simulink model "helicopter_2DOF"  (R2026a)
settings: Solver=VariableStepAuto  StopTime=25
values from neighbouring files (symbols this model uses):
  act = getBaseVariable('act')    [run_simulink_simulations.m]
  aero = struct    [run_simulink_simulations.m]
  alpha0 = deg2rad(15)    [build_uncertain_linear_model.m]    (also in init.m; run_simulink_simulations.m = evalin('base','alpha0'))
  Aobs = A - Ke*Cmeas    [LQG_2DOF_Synthesis.m]    (also in PIDcomp_decoupler_sensitivity.m; run_simulink_simulations.m)
  beta0 = deg2rad(20)    [build_uncertain_linear_model.m]    (also in init.m; run_simulink_simulations.m = evalin('base','beta0'))
  Bobs = [B Ke]    [LQG_2DOF_Synthesis.m]    (also in PIDcomp_decoupler_sensitivity.m; run_simulink_simulations.m)
  Cobs = eye(size(A))    [LQG_2DOF_Synthesis.m]    (also in PIDcomp_decoupler_sensitivity.m; run_simulink_simulations.m)
  Ddec_phys = [0.00367730883727  -0.0180750563026; -0.000204187403773  0.138403763822]    [HINF_controllers.mat]    (also in HINF_synthesis.m = Du *      Ddec_scaled *      Du_inv)
  delta_plant = zeros(7,1)    [init.m]
  denFalpha = [1 28.9710633828]    [HINF_controllers.mat]
  denFbeta = [1 116.132169803]    [HINF_controllers.mat]
  Dobs = zeros(size(A,1), size(B,2) + size(Cmeas,1))    [LQG_2DOF_Synthesis.m]    (also in PIDcomp_decoupler_sensitivity.m = zeros(size(A,1),size(B,2)+size(Cmeas,1)); run_simulink_simulations.m = zeros(size(A,1),size(B,2)+size(Cmeas,1)))
  g = 9.81    [build_uncertain_linear_model.m]
  HINF_controller_id = 3    [init.m]
  Hy = (Jsensor.'*Vinv*Jsensor) \      (Jsensor.'*Vinv)    [HINF_setup.m]    (also in HINF_setup.mat = [0.105532740103  0  0; 0  -0.00735527189948  -0.020208443457; RAS_vectorized.m = (Jsensor.'*Vinv*Jsensor) \ (Jsensor.'*Vinv))
  Hy_LQG = [0.105532740103  0  0; 0  -0.00735527189948  -0.0202084434578]    [LQG_2DOF_Controllers.mat]    (also in LQG_2DOF_Synthesis.m = (Jsensor.'*Vinv*Jsensor) \      (Jsensor.'*Vinv))
  K_hinfsyn = minreal(          Du *          K_hinfsyn_scaled *          Dy_inv,          1e-7)    [HINF_synthesis.m]
  K_LQG = ss(      Ac_LQG,      Bc_LQG,      Cc_LQG,      Dc_LQG)    [LQG_2DOF_Synthesis.m]
  K_mix = minreal(          Du *          K_mix_scaled *          Dy_inv,          1e-7)    [HINF_synthesis.m]
  K_mu = minreal(          Du *          K_mu_scaled *          Dy_inv,          1e-7)    [MU_synthesis.m]
  Kalpha_tuned = pid(          alphaScaledToPhys *          Kalpha_tuned_scaled.Kp,          alphaScaledToPhys *          Kalpha_tuned_scaled.Ki,          alphaScaledToPhys *          Kalpha_tuned_scaled.Kd,          Kalpha_tuned_scaled.Tf)    [HINF_synthesis.m]
  Kbeta_tuned = pid(          betaScaledToPhys *          Kbeta_tuned_scaled.Kp,          betaScaledToPhys *          Kbeta_tuned_scaled.Ki,          betaScaledToPhys *          Kbeta_tuned_scaled.Kd,          Kbeta_tuned_scaled.Tf)    [HINF_synthesis.m]
  Ki_LQGI = [-6.12353410994  -0.048270119194; 0.0482701191938  -6.12353410994]    [LQG_2DOF_Controllers.mat]    (also in LQG_2DOF_Synthesis.m = Kaug_LQI(:,n+1:end))
  Kx_LQGI = [2.67945787682 0.0236091239115 4.27147445601 0.0421494721099 7.37552374356 0.124215129254 0.0236091239115 3.00325151028 0.0375549932522 4.81803854156 0.0741131674737 8.79398804244 ... (20 elements, 2x10)]    [LQG_2DOF_Controllers.mat]    (also in LQG_2DOF_Synthesis.m = Kaug_LQI(:,1:n))
  LQG_controller_id = 1    [init.m]
  LQG_plant_id = 1    [init.m]
  numFalpha = [5.51938404497 96.5040578252]    [HINF_controllers.mat]
  numFbeta = [0.20657402382 68.2554624776]    [HINF_controllers.mat]
  P_nominal_ext = ss(P_uncertain_ext.NominalValue)    [build_uncertain_linear_model.m]
  q0 = [alpha0; beta0]    [init.m]
  qdot0 = [0; 0]    [init.m]
  ref = struct    [run_simulink_simulations.m]
  Robust_plant_id = 2    [init.m]
  sensor = getBaseVariable('sensor')    [run_simulink_simulations.m]
  u0 = u0_nominal    [build_uncertain_linear_model.m]    (also in init.m = E0 \ [)
  x0 = [ ... (first row only)    [build_uncertain_linear_model.m]    (also in init.m = [alpha0; 0; beta0; 0])
  xhat0 = zeros(size(A,1),1)    [LQG_2DOF_Synthesis.m]    (also in PIDcomp_decoupler_sensitivity.m; run_simulink_simulations.m)
  y0_sensor = [ ... (first row only)    [HINF_setup.m]    (also in HINF_setup.mat = [2.53901483246 43.6957068665 -15.9039366646]; LQG_2DOF_Controllers.mat = [2.53901483246 43.6957068665 -15.9039366646]; LQG_2DOF_Synthesis.m; RAS_vectorized.m)
undefined symbols (not defined in the file or in its folder): params
libraries: simulink x4, slpidlib x2, cstblocks_lti x2, RCTblocks x2
settings Model: Creator=bonci  LastModifiedBy=giggi
settings DebuggingCC: UnderSpecifiedDimensionMsg=warning

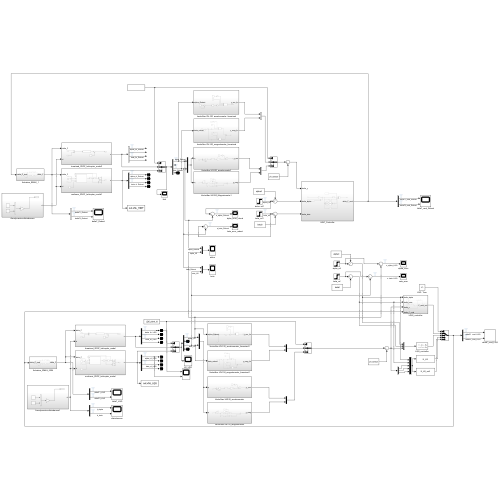
[thumbnail: Simulink's stored preview of the top-level diagram]
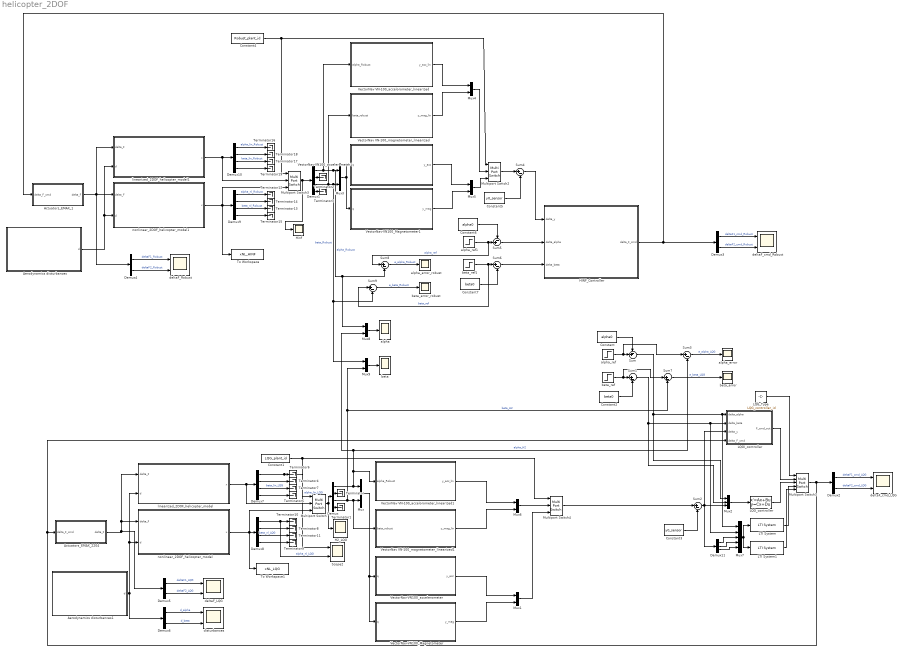
== system helicopter_2DOF ==
  Actuators_EMAX_1 : Subsystem
  Actuators_EMAX_2204 : Subsystem
  Aerodynamics disturbances : Subsystem
  Aerodynamics disturbances1 : Subsystem
  Constant : Constant  Value=alpha0
  Constant1 : Constant  Value=LQG_plant_id
  Constant2 : Constant  Value=beta0
  Constant3 : Constant  Value=y0_sensor
  Constant4 : Constant  Value=Robust_plant_id
  Constant5 : Constant  Value=y0_sensor
  Constant6 : Constant  Value=alpha0
  Constant7 : Constant  Value=beta0
  Demux{,1,7..10} (6 alike) : Demux
  Demux11 : Demux  Outputs=3
  Demux{2..6} (5 alike) : Demux  Outputs=2
  H2_LQG : Scope
      settings: ActiveDisplayYMinimum=0.24953416869226661  ActiveDisplayYMaximum=0.36288471920080412
  HINF_Controller : Subsystem
  Hinf : Scope
      settings: ActiveDisplayYMinimum=0.24925633700219857  ActiveDisplayYMaximum=0.36252454674659934
  LQGI_controller : Subsystem
  LQG_Type : Constant  Value=LQG_controller_id
  LQG_controller : StateSpace  A=K_LQG.A  B=K_LQG.B  C=K_LQG.C  D=K_LQG.D  InitialCondition=zeros(size(K_LQG.A,1),1)
  LTI System : cstblocks_lti/LTI System  sys=K_H2  IC=[]  PadeOrder=0
      settings: LibrarySourceBlock=cstblocks/LTI System
  LTI System1 : cstblocks_lti/LTI System  sys=K_H2_soft  IC=[]  PadeOrder=0
      settings: LibrarySourceBlock=cstblocks/LTI System
  Multiport Switch{,2..4} (4 alike) : MultiPortSwitch  Inputs=2  SaturateOnIntegerOverflow=off  InputSameDT=off
  Multiport Switch1 : MultiPortSwitch  Inputs=4  SaturateOnIntegerOverflow=off  InputSameDT=off
  Mux{,1,3..6,8..9} (8 alike) : Mux  Inputs=2
  Mux2 : Mux  Inputs=3
  Mux7 : Mux  Inputs=5
  Scope2 : Scope  NumInputPorts=2
      settings: ActiveDisplayYMinimum=0.25286399867414605  ActiveDisplayYMaximum=0.34221788992417967  DataLoggingVariableName=ScopeData11
  Sum : Sum  Inputs=-+|
  Sum{1..4,6..9} (8 alike) : Sum  Inputs=|+-
  Sum5 : Sum  Inputs=-+|
  Terminator{,1..19} (20 alike) : Terminator
  To Workspace : ToWorkspace  VariableName=xNL_HINF  SaveFormat=Timeseries  SampleTime=-1
  To Workspace1 : ToWorkspace  VariableName=xNL_LQG  SaveFormat=Timeseries  SampleTime=-1
  VectorNav VN-100_accelorometer_linearized : Subsystem
  VectorNav VN-100_accelorometer_linearized1 : Subsystem
  VectorNav VN-100_magnetometer_linearized : Subsystem
  VectorNav VN-100_magnetometer_linearized1 : Subsystem
  VectorNav-VN100_Magnetometer : Subsystem
  VectorNav-VN100_Magnetometer1 : Subsystem
  VectorNav-VN100_accelerometer : Subsystem
  VectorNav-VN100_accelerometer1 : Subsystem
  alpha : Scope
      settings: ActiveDisplayYMinimum=0.25090839242771618  ActiveDisplayYMaximum=0.2720900672525749  DataLoggingVariableName=ScopeData12
  alpha_error : Scope
      settings: DataLoggingVariableName=ScopeData2
  alpha_error_robust : Scope
      settings: DataLoggingVariableName=ScopeData4
  alpha_ref : Step  Time=ref.alpha.time  InitialValue=ref.alpha.initial  FinalValue=ref.alpha.final  SampleTime=0
  alpha_ref1 : Step  Time=ref.alpha.time  InitialValue=ref.alpha.initial  FinalValue=ref.alpha.final  SampleTime=0
  beta : Scope
      settings: ActiveDisplayYMinimum=0.33140553496326319  ActiveDisplayYMaximum=0.36028063841557784  DataLoggingVariableName=ScopeData13
  beta_error : Scope
      settings: ActiveDisplayYMinimum=-0.017727079570451457  ActiveDisplayYMaximum=0.0030981168879630895  DataLoggingVariableName=ScopeData3
  beta_error_robust : Scope
      settings: DataLoggingVariableName=ScopeData5
  beta_ref : Step  Time=ref.beta.time  InitialValue=ref.beta.initial  FinalValue=ref.beta.final  SampleTime=0
  beta_ref1 : Step  Time=ref.beta.time  InitialValue=ref.beta.initial  FinalValue=ref.beta.final  SampleTime=0
  deltaF_LQG : Scope  NumInputPorts=2
      settings: DataLoggingVariableName=ScopeData9
  deltaF_Robust : Scope  NumInputPorts=2
      settings: DataLoggingVariableName=ScopeData8
  deltaF_cmd_LQG : Scope  NumInputPorts=2
      settings: ActiveDisplayYMinimum=-6.7119063745859271E-6  ActiveDisplayYMaximum=6.008697179895143E-5  DataLoggingVariableName=ScopeData6
  deltaF_cmd_Robust : Scope  NumInputPorts=2
      settings: ActiveDisplayYMinimum=-5.0521969284629318E-5  ActiveDisplayYMaximum=0.00043770968760487613  DataLoggingVariableName=ScopeData7
  disturbances : Scope  NumInputPorts=2
      settings: DataLoggingVariableName=ScopeData10
  linearized_2DOF_helicopter_model : Subsystem
  linearized_2DOF_helicopter_model1 : Subsystem
  nonlinear_2DOF_helicopter_model : Subsystem
  nonlinear_2DOF_helicopter_model1 : Subsystem
  wires:
  nonlinear_2DOF_helicopter_model/1(x) -> Demux8/1, To Workspace1/1, Multiport Switch/3
  linearized_2DOF_helicopter_model/1(x) -> Multiport Switch/2, Demux7/1
  Constant1/1 -> Multiport Switch4/1, Multiport Switch/1
  Multiport Switch/1 -> Demux/1, H2_LQG/1
  VectorNav-VN100_accelerometer/1(y_acc) -> Mux1/1
  VectorNav-VN100_Magnetometer/1(y_mag) -> Mux1/2
  Demux/1 -> VectorNav VN-100_accelorometer_linearized1/1(alpha_Robust), Sum3/2, Mux8/2, Mux/1  "alpha_H2"
  Demux/3 -> Mux9/2, Sum7/2, VectorNav VN-100_magnetometer_linearized1/1(bata_robust), Mux/2  "beta_H2"
  Mux/1 -> VectorNav-VN100_Magnetometer/1(q), VectorNav-VN100_accelerometer/1(q)
  Demux/2 -> Terminator/1
  Demux/4 -> Terminator1/1
  alpha_ref/1 -> Sum3/1, Sum/2
  beta_ref/1 -> Sum7/1, Sum1/1
  Constant/1 -> Sum/1
  Constant2/1 -> Sum1/2
  Constant3/1 -> Sum2/2
  Sum/1 -> Mux7/1, LQGI_controller/1(delta_alpha), Mux2/1
  Mux2/1 -> LQG_controller/1
  LQG_controller/1 -> Multiport Switch1/3
  LQG_Type/1 -> Multiport Switch1/1
  Multiport Switch1/1 -> LQGI_controller/4(delta_F_cmd), Actuators_EMAX_2204/1(delta_F_cmd), Demux2/1
  LQGI_controller/1(F_cmd_out) -> Multiport Switch1/2
  Constant5/1 -> Sum4/2
  VectorNav-VN100_accelerometer1/1(y_acc) -> Mux5/1
  Demux1/1 -> VectorNav VN-100_accelorometer_linearized/1(alpha_Robust), Mux8/1, Sum8/2, Mux3/1  "alpha_Robust"
  VectorNav-VN100_Magnetometer1/1(y_mag) -> Mux5/2
  Mux3/1 -> VectorNav-VN100_Magnetometer1/1(q), VectorNav-VN100_accelerometer1/1(q)
  Demux1/2 -> Terminator2/1
  Demux1/4 -> Terminator3/1
  Demux1/3 -> VectorNav VN-100_magnetometer_linearized/1(bata_robust), Mux3/2, Mux9/1, Sum9/2  "beta_Robust"
  Constant4/1 -> Multiport Switch3/1, Multiport Switch2/1
  Multiport Switch3/1 -> Demux1/1, Hinf/1
  linearized_2DOF_helicopter_model1/1(x) -> Demux10/1, Multiport Switch3/2
  Constant6/1 -> Sum5/1
  alpha_ref1/1 -> Sum8/1, Sum5/2  "alpha_ref"
  beta_ref1/1 -> Sum9/1, Sum6/1  "beta_ref"
  Constant7/1 -> Sum6/2
  Sum4/1 -> HINF_Controller/1(delta_y)
  Sum5/1 -> HINF_Controller/2(delta_alpha)
  Sum6/1 -> HINF_Controller/3(delta_beta)
  Aerodynamics disturbances/1(d) -> linearized_2DOF_helicopter_model1/2(d), nonlinear_2DOF_helicopter_model1/2(d)
  Sum3/1 -> alpha_error/1  "e_alpha_LQG"
  Sum1/1 -> LQGI_controller/2(delta_beta), Mux7/2, Mux2/2
  Sum7/1 -> beta_error/1  "e_beta_LQG"
  Sum8/1 -> alpha_error_robust/1  "e_alpha_Robust"
  Sum9/1 -> beta_error_robust/1  "e_beta_Robust"
  Demux2/1 -> deltaF_cmd_LQG/1  "deltaF1_cmd_LQG"
  Demux2/2 -> deltaF_cmd_LQG/2  "deltaF2_cmd_LQG"
  Demux3/2 -> deltaF_cmd_Robust/2  "deltaF2_cmd_Robust"
  Demux3/1 -> deltaF_cmd_Robust/1  "deltaF1_cmd_Robust"
  HINF_Controller/1(delta_F_cmd) -> Demux3/1, Actuators_EMAX_1/1(delta_F_cmd)
  Actuators_EMAX_1/1(delta_F) -> nonlinear_2DOF_helicopter_model1/1(delta_F), linearized_2DOF_helicopter_model1/1(delta_F), Demux4/1
  Demux4/1 -> deltaF_Robust/1  "deltaF1_Robust"
  Demux4/2 -> deltaF_Robust/2  "deltaF2_Robust"
  Demux5/1 -> deltaF_LQG/1  "deltaF1_LQG"
  Demux5/2 -> deltaF_LQG/2  "deltaF2_LQG"
  Actuators_EMAX_2204/1(delta_F) -> Demux5/1, nonlinear_2DOF_helicopter_model/1(delta_F), linearized_2DOF_helicopter_model/1(delta_F)
  Demux6/2 -> disturbances/2  "d_beta"
  Aerodynamics disturbances1/1(d) -> Demux6/1, nonlinear_2DOF_helicopter_model/2(d), linearized_2DOF_helicopter_model/2(d)
  Demux6/1 -> disturbances/1  "d_alpha"
  Demux7/4 -> Terminator5/1
  Demux7/1 -> Scope2/1, Terminator6/1  "alpha_lin_LQG"
  Demux7/3 -> Terminator7/1  "beta_lin_LQG"
  Demux7/2 -> Terminator4/1
  Demux8/1 -> Scope2/2, Terminator10/1  "alpha_nl_LQG"
  Demux8/2 -> Terminator8/1
  Demux8/3 -> Terminator11/1  "beta_nl_LQG"
  Demux8/4 -> Terminator9/1
  Demux9/4 -> Terminator15/1
  Demux9/3 -> Terminator13/1  "beta_nl_Robust"
  nonlinear_2DOF_helicopter_model1/1(x) -> Demux9/1, To Workspace/1, Multiport Switch3/3
  Demux9/1 -> Terminator12/1  "alpha_nl_Robust"
  Demux9/2 -> Terminator14/1
  Demux10/3 -> Terminator17/1  "beta_lin_Robust"
  Demux10/4 -> Terminator19/1
  Demux10/1 -> Terminator16/1  "alpha_lin_Robust"
  Demux10/2 -> Terminator18/1
  Mux5/1 -> Multiport Switch2/3
  Multiport Switch2/1 -> Sum4/1
  Mux1/1 -> Multiport Switch4/3
  Multiport Switch4/1 -> Sum2/1
  VectorNav VN-100_magnetometer_linearized/1(y_mag_lin) -> Mux4/2
  VectorNav VN-100_accelorometer_linearized/1(y_acc_lin) -> Mux4/1
  Mux4/1 -> Multiport Switch2/2
  VectorNav VN-100_accelorometer_linearized1/1(y_acc_lin) -> Mux6/1
  VectorNav VN-100_magnetometer_linearized1/1(y_mag_lin) -> Mux6/2
  Mux6/1 -> Multiport Switch4/2
  Sum2/1 -> Demux11/1, LQGI_controller/3(delta_y), Mux2/3
  Demux11/1 -> Mux7/3
  Demux11/2 -> Mux7/4
  Demux11/3 -> Mux7/5
  Mux7/1 -> LTI System1/1, LTI System/1
  LTI System/1 -> Multiport Switch1/4
  LTI System1/1 -> Multiport Switch1/5
  Mux8/1 -> alpha/1
  Mux9/1 -> beta/1

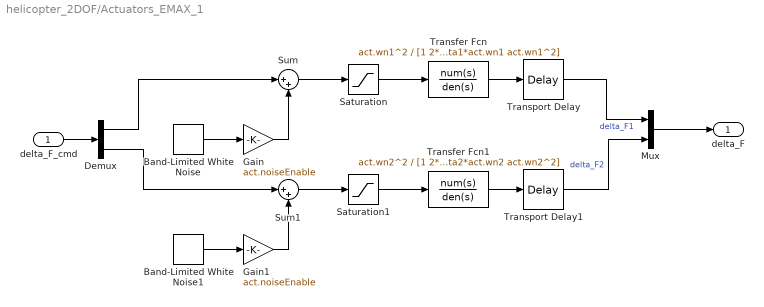
== system helicopter_2DOF/Actuators_EMAX_1 ==
  delta_F_cmd : Inport
  Band-Limited White Noise : simulink/Sources/Band-Limited White Noise  Cov=act.noisePower_F1  Ts=act.Ts_noise  seed=act.seed
  Band-Limited White Noise1 : simulink/Sources/Band-Limited White Noise  Cov=act.noisePower_F2  Ts=act.Ts_noise  seed=act.seed+1
  Demux : Demux  Outputs=2
  Gain : Gain  Gain=act.noiseEnable
  Gain1 : Gain  Gain=act.noiseEnable
  Mux : Mux  Inputs=2
  Saturation : Saturate  UpperLimit=act.deltaF1_max  LowerLimit=act.deltaF1_min
  Saturation1 : Saturate  UpperLimit=act.deltaF2_max  LowerLimit=act.deltaF2_min
  Sum : Sum  Inputs=|++
  Sum1 : Sum  Inputs=|++
  Transfer Fcn : TransferFcn  Numerator=act.wn1^2  Denominator=[1 2*act.zeta1*act.wn1 act.wn1^2]
  Transfer Fcn1 : TransferFcn  Numerator=act.wn2^2  Denominator=[1 2*act.zeta2*act.wn2 act.wn2^2]
  Transport Delay : TransportDelay  DelayTime=act.td1
  Transport Delay1 : TransportDelay  DelayTime=act.td2
  delta_F : Outport
  wires:
  Gain/1 -> Sum/2
  Saturation1/1 -> Transfer Fcn1/1
  Sum/1 -> Saturation/1
  Mux/1 -> delta_F/1
  Demux/1 -> Sum/1
  Transport Delay/1 -> Mux/1  "delta_F1"
  Transfer Fcn/1 -> Transport Delay/1
  Demux/2 -> Sum1/1
  Transfer Fcn1/1 -> Transport Delay1/1
  Band-Limited White Noise1/1 -> Gain1/1
  Gain1/1 -> Sum1/2
  Sum1/1 -> Saturation1/1
  Transport Delay1/1 -> Mux/2  "delta_F2"
  delta_F_cmd/1 -> Demux/1
  Band-Limited White Noise/1 -> Gain/1
  Saturation/1 -> Transfer Fcn/1

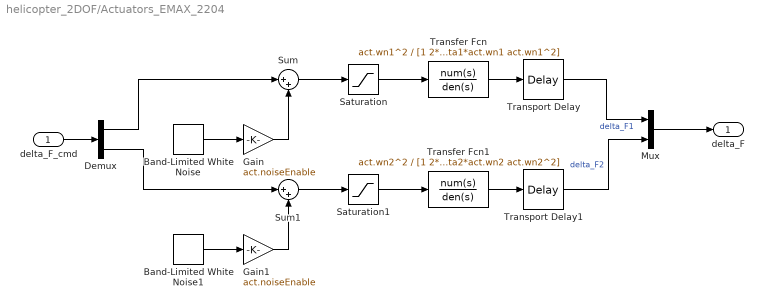
== system helicopter_2DOF/Actuators_EMAX_2204 ==
  delta_F_cmd : Inport
  Band-Limited White Noise : simulink/Sources/Band-Limited White Noise  Cov=act.noisePower_F1  Ts=act.Ts_noise  seed=act.seed
  Band-Limited White Noise1 : simulink/Sources/Band-Limited White Noise  Cov=act.noisePower_F2  Ts=act.Ts_noise  seed=act.seed + 1
  Demux : Demux  Outputs=2
  Gain : Gain  Gain=act.noiseEnable
  Gain1 : Gain  Gain=act.noiseEnable
  Mux : Mux  Inputs=2
  Saturation : Saturate  UpperLimit=act.deltaF1_max  LowerLimit=act.deltaF1_min
  Saturation1 : Saturate  UpperLimit=act.deltaF2_max  LowerLimit=act.deltaF2_min
  Sum : Sum  Inputs=|++
  Sum1 : Sum  Inputs=|++
  Transfer Fcn : TransferFcn  Numerator=act.wn1^2  Denominator=[1 2*act.zeta1*act.wn1 act.wn1^2]
  Transfer Fcn1 : TransferFcn  Numerator=act.wn2^2  Denominator=[1 2*act.zeta2*act.wn2 act.wn2^2]
  Transport Delay : TransportDelay  DelayTime=act.td1
  Transport Delay1 : TransportDelay  DelayTime=act.td2
  delta_F : Outport
  wires:
  Gain/1 -> Sum/2
  Saturation1/1 -> Transfer Fcn1/1
  Sum/1 -> Saturation/1
  Mux/1 -> delta_F/1
  Demux/1 -> Sum/1
  Transport Delay/1 -> Mux/1  "delta_F1"
  Transfer Fcn/1 -> Transport Delay/1
  Demux/2 -> Sum1/1
  Transfer Fcn1/1 -> Transport Delay1/1
  Band-Limited White Noise1/1 -> Gain1/1
  Gain1/1 -> Sum1/2
  Sum1/1 -> Saturation1/1
  Transport Delay1/1 -> Mux/2  "delta_F2"
  delta_F_cmd/1 -> Demux/1
  Band-Limited White Noise/1 -> Gain/1
  Saturation/1 -> Transfer Fcn/1

== system helicopter_2DOF/Aerodynamics disturbances ==
  Gain : Gain  Gain=aero.enable
  Mux3 : Mux  Inputs=2
  Step : Step  Time=aero.alpha.time  FinalValue=aero.alpha.amplitude  SampleTime=0
  Step1 : Step  Time=aero.beta.time  FinalValue=aero.beta.amplitude  SampleTime=0
  d : Outport
  wires:
  Step/1 -> Mux3/1
  Mux3/1 -> Gain/1
  Step1/1 -> Mux3/2
  Gain/1 -> d/1

== system helicopter_2DOF/Aerodynamics disturbances1 ==
  Gain : Gain  Gain=aero.enable
  Mux3 : Mux  Inputs=2
  Step : Step  Time=aero.alpha.time  FinalValue=aero.alpha.amplitude  SampleTime=0
  Step1 : Step  Time=aero.beta.time  FinalValue=aero.beta.amplitude  SampleTime=0
  d : Outport
  wires:
  Step/1 -> Mux3/1
  Mux3/1 -> Gain/1
  Step1/1 -> Mux3/2
  Gain/1 -> d/1

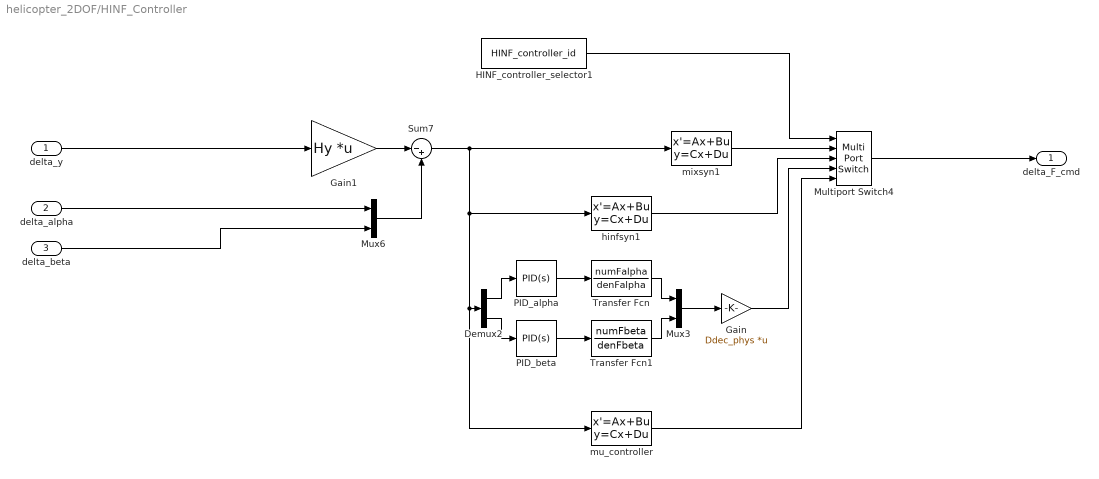
== system helicopter_2DOF/HINF_Controller ==
  delta_y : Inport
  delta_alpha : Inport  Port=2
  delta_beta : Inport  Port=3
  Demux2 : Demux  Outputs=2
  Gain : Gain  Gain=Ddec_phys  Multiplication=Matrix(K*u)
  Gain1 : Gain  Gain=Hy  Multiplication=Matrix(K*u)
  HINF_controller_selector1 : Constant  Value=HINF_controller_id
  Multiport Switch4 : MultiPortSwitch  Inputs=4  SaturateOnIntegerOverflow=off  InputSameDT=off
  Mux3 : Mux  Inputs=2
  Mux6 : Mux  Inputs=2
  PID_alpha : slpidlib/PID Controller  Controller=PID  Form=Parallel  TimeDomain=Continuous-time  UseExternalTs=off  SampleTime=-1  IntegratorMethod=Forward Euler  FilterMethod=Forward Euler  ControllerParametersSource=internal  P=Kalpha_tuned.Kp  I=Kalpha_tuned.Ki  UseKiTs=off  D=Kalpha_tuned.Kd  UseExternalDerivativeSource=off  N=1/Kalpha_tuned.Tf  UseFilter=on  TunerSelectOption=Transfer Function Based (PID Tuner App)  InitialConditionSource=internal  InitialConditionForIntegrator=0  InitialConditionForFilter=0  DifferentiatorICPrevScaledInput=0  ExternalReset=none  TrackingMode=off  Kt=1  LimitOutput=off  SatLimitsSource=internal  UpperSaturationLimit=inf  LowerSaturationLimit=-inf  LinearizeAsGain=on  AntiWindupMode=none  Kb=1  LimitIntegrator=off  UpperIntegratorSaturationLimit=inf  LowerIntegratorSaturationLimit=-inf  POutMin=[]  POutMax=[]  IOutMin=[]  IOutMax=[]  DOutMin=[]  DOutMax=[]  NOutMin=[]  NOutMax=[]  SumOutMin=[]  SumOutMax=[]  SaturationOutMin=[]  SaturationOutMax=[]  PParamMin=[]  PParamMax=[]  IParamMin=[]  IParamMax=[]  DParamMin=[]  DParamMax=[]  NParamMin=[]  NParamMax=[]  KbParamMin=[]  KbParamMax=[]  KtParamMin=[]  KtParamMax=[]  KbOutMin=[]  KbOutMax=[]  KtOutMin=[]  KtOutMax=[]  IntegratorOutMin=[]  IntegratorOutMax=[]  FilterOutMin=[]  FilterOutMax=[]  SumI1OutMin=[]  SumI1OutMax=[]  SumI2OutMin=[]  SumI2OutMax=[]  SumI3OutMin=[]  SumI3OutMax=[]  SumI4OutMin=[]  SumI4OutMax=[]  SumDOutMin=[]  SumDOutMax=[]  DifferentiatorOutMin=[]  DifferentiatorOutMax=[]  FilterDiffOutCoefMin=[]  FilterDiffOutCoefMax=[]  ReciprocalOutMin=[]  ReciprocalOutMax=[]  SumDenOutMin=[]  SumDenOutMax=[]  SumNumOutMin=[]  SumNumOutMax=[]  DivideOutMin=[]  DivideOutMax=[]  UdiffTsProdOutMin=[]  UdiffTsProdOutMax=[]  NTsProdOutMin=[]  NTsProdOutMax=[]  UintegralTsProdOutMin=[]  UintegralTsProdOutMax=[]  UngainTsProdOutMin=[]  UngainTsProdOutMax=[]  ClampingZeroOutDataTypeStr=Inherit: Inherit via back propagation  ClampingZeroOutMin=[]  ClampingZeroOutMax=[]  FilterDenConstantOutDataTypeStr=Inherit: Inherit via back propagation  FilterDenConstantOutMin=[]  FilterDenConstantOutMax=[]  PCopyOutDataTypeStr=Inherit: Inherit via back propagation  PCopyOutMin=[]  PCopyOutMax=[]  NCopyOutDataTypeStr=Inherit: Inherit via back propagation  NCopyOutMin=[]  NCopyOutMax=[]  IntegratorContinuousStateAttributes=''  IntegratorStateMustResolveToSignalObject=off  IntegratorRTWStateStorageClass=Auto  FilterContinuousStateAttributes=''  FilterStateMustResolveToSignalObject=off  FilterRTWStateStorageClass=Auto  ParallelPVariant=InternalParameters  IdealPVariant=Disabled  IVariant=InternalParameters  DVariant=InternalParameters  IntegratorVariant=Continuous  SatVariant=Disabled  AWVariant=Passthrough  PCopyVariant=Disabled  TRVariant=Disabled  FdbkBlocksVariant=Forward  IdealPFdbkVariant=Disabled  SatFdbkVariant=Disabled  DerivativeFilterVariant=ContFilter  NVariant=InternalParameters  NCopyVariant=Disabled  FilterICVariant=InternalICsFilter  IntegratorICVariant=InternalICs  ExternalResetVariant=Disabled  TRSumVariant=Passthrough  SumFdbkVariant=Disabled  SumVariant=Sum_PID  TsampFilterVariant=InternalTs  TsampNgainVariant=Passthrough  TsampIntegralVariant=Disabled_SignalSpec  ExternalSaturationOutDataTypeStr=Inherit: Same as second input  DerivativeSourceVariant=ErrorSignal  PreIntVariant=InternalPreInt
  PID_beta : slpidlib/PID Controller  Controller=PID  Form=Parallel  TimeDomain=Continuous-time  UseExternalTs=off  SampleTime=-1  IntegratorMethod=Forward Euler  FilterMethod=Forward Euler  ControllerParametersSource=internal  P=Kbeta_tuned.Kp  I=Kbeta_tuned.Ki  UseKiTs=off  D=Kbeta_tuned.Kd  UseExternalDerivativeSource=off  N=1/Kbeta_tuned.Tf  UseFilter=on  TunerSelectOption=Transfer Function Based (PID Tuner App)  InitialConditionSource=internal  InitialConditionForIntegrator=0  InitialConditionForFilter=0  DifferentiatorICPrevScaledInput=0  ExternalReset=none  TrackingMode=off  Kt=1  LimitOutput=off  SatLimitsSource=internal  UpperSaturationLimit=inf  LowerSaturationLimit=-inf  LinearizeAsGain=on  AntiWindupMode=none  Kb=1  LimitIntegrator=off  UpperIntegratorSaturationLimit=inf  LowerIntegratorSaturationLimit=-inf  POutMin=[]  POutMax=[]  IOutMin=[]  IOutMax=[]  DOutMin=[]  DOutMax=[]  NOutMin=[]  NOutMax=[]  SumOutMin=[]  SumOutMax=[]  SaturationOutMin=[]  SaturationOutMax=[]  PParamMin=[]  PParamMax=[]  IParamMin=[]  IParamMax=[]  DParamMin=[]  DParamMax=[]  NParamMin=[]  NParamMax=[]  KbParamMin=[]  KbParamMax=[]  KtParamMin=[]  KtParamMax=[]  KbOutMin=[]  KbOutMax=[]  KtOutMin=[]  KtOutMax=[]  IntegratorOutMin=[]  IntegratorOutMax=[]  FilterOutMin=[]  FilterOutMax=[]  SumI1OutMin=[]  SumI1OutMax=[]  SumI2OutMin=[]  SumI2OutMax=[]  SumI3OutMin=[]  SumI3OutMax=[]  SumI4OutMin=[]  SumI4OutMax=[]  SumDOutMin=[]  SumDOutMax=[]  DifferentiatorOutMin=[]  DifferentiatorOutMax=[]  FilterDiffOutCoefMin=[]  FilterDiffOutCoefMax=[]  ReciprocalOutMin=[]  ReciprocalOutMax=[]  SumDenOutMin=[]  SumDenOutMax=[]  SumNumOutMin=[]  SumNumOutMax=[]  DivideOutMin=[]  DivideOutMax=[]  UdiffTsProdOutMin=[]  UdiffTsProdOutMax=[]  NTsProdOutMin=[]  NTsProdOutMax=[]  UintegralTsProdOutMin=[]  UintegralTsProdOutMax=[]  UngainTsProdOutMin=[]  UngainTsProdOutMax=[]  ClampingZeroOutDataTypeStr=Inherit: Inherit via back propagation  ClampingZeroOutMin=[]  ClampingZeroOutMax=[]  FilterDenConstantOutDataTypeStr=Inherit: Inherit via back propagation  FilterDenConstantOutMin=[]  FilterDenConstantOutMax=[]  PCopyOutDataTypeStr=Inherit: Inherit via back propagation  PCopyOutMin=[]  PCopyOutMax=[]  NCopyOutDataTypeStr=Inherit: Inherit via back propagation  NCopyOutMin=[]  NCopyOutMax=[]  IntegratorContinuousStateAttributes=''  IntegratorStateMustResolveToSignalObject=off  IntegratorRTWStateStorageClass=Auto  FilterContinuousStateAttributes=''  FilterStateMustResolveToSignalObject=off  FilterRTWStateStorageClass=Auto  ParallelPVariant=InternalParameters  IdealPVariant=Disabled  IVariant=InternalParameters  DVariant=InternalParameters  IntegratorVariant=Continuous  SatVariant=Disabled  AWVariant=Passthrough  PCopyVariant=Disabled  TRVariant=Disabled  FdbkBlocksVariant=Forward  IdealPFdbkVariant=Disabled  SatFdbkVariant=Disabled  DerivativeFilterVariant=ContFilter  NVariant=InternalParameters  NCopyVariant=Disabled  FilterICVariant=InternalICsFilter  IntegratorICVariant=InternalICs  ExternalResetVariant=Disabled  TRSumVariant=Passthrough  SumFdbkVariant=Disabled  SumVariant=Sum_PID  TsampFilterVariant=InternalTs  TsampNgainVariant=Passthrough  TsampIntegralVariant=Disabled_SignalSpec  ExternalSaturationOutDataTypeStr=Inherit: Same as second input  DerivativeSourceVariant=ErrorSignal  PreIntVariant=InternalPreInt
  Sum7 : Sum  Inputs=|-+
  Transfer Fcn : TransferFcn  Numerator=numFalpha  Denominator=denFalpha
  Transfer Fcn1 : TransferFcn  Numerator=numFbeta  Denominator=denFbeta
  hinfsyn1 : StateSpace  A=K_hinfsyn.A  B=K_hinfsyn.B  C=K_hinfsyn.C  D=K_hinfsyn.D  InitialCondition=zeros(size(K_hinfsyn.A,1),1)
  mixsyn1 : StateSpace  A=K_mix.A  B=K_mix.B  C=K_mix.C  D=K_mix.D  InitialCondition=zeros(size(K_mix.A,1),1)
  mu_controller : StateSpace  A=K_mu.A  B=K_mu.B  C=K_mu.C  D=K_mu.D  InitialCondition=zeros(size(K_mu.A,1),1)
  delta_F_cmd : Outport
  wires:
  Gain1/1 -> Sum7/1
  Sum7/1 -> mixsyn1/1, hinfsyn1/1, mu_controller/1, Demux2/1
  Mux6/1 -> Sum7/2
  mixsyn1/1 -> Multiport Switch4/2
  HINF_controller_selector1/1 -> Multiport Switch4/1
  PID_alpha/1 -> Transfer Fcn/1
  hinfsyn1/1 -> Multiport Switch4/3
  delta_y/1 -> Gain1/1
  delta_alpha/1 -> Mux6/1
  Multiport Switch4/1 -> delta_F_cmd/1
  delta_beta/1 -> Mux6/2
  Mux3/1 -> Gain/1
  Transfer Fcn/1 -> Mux3/1
  Transfer Fcn1/1 -> Mux3/2
  PID_beta/1 -> Transfer Fcn1/1
  Demux2/1 -> PID_alpha/1
  Demux2/2 -> PID_beta/1
  mu_controller/1 -> Multiport Switch4/5
  Gain/1 -> Multiport Switch4/4

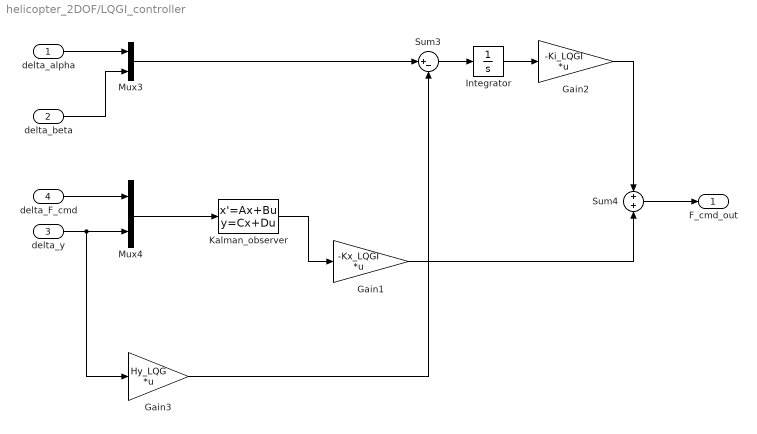
== system helicopter_2DOF/LQGI_controller ==
  delta_alpha : Inport
  delta_beta : Inport  Port=2
  delta_y : Inport  Port=3
  delta_F_cmd : Inport  Port=4
  Gain1 : Gain  Gain=-Kx_LQGI  Multiplication=Matrix(K*u)
  Gain2 : Gain  Gain=-Ki_LQGI  Multiplication=Matrix(K*u)
  Gain3 : Gain  Gain=Hy_LQG  Multiplication=Matrix(K*u)
  Integrator : Integrator  InitialCondition=zeros(2,1)
  Kalman_observer : StateSpace  A=Aobs  B=Bobs  C=Cobs  D=Dobs  InitialCondition=xhat0
  Mux3 : Mux  Inputs=2
  Mux4 : Mux  Inputs=2
  Sum3 : Sum  Inputs=|+-
  Sum4 : Sum  Inputs=+|+
  F_cmd_out : Outport
  wires:
  Gain2/1 -> Sum4/1
  Mux3/1 -> Sum3/1
  Sum3/1 -> Integrator/1
  Gain1/1 -> Sum4/2
  Kalman_observer/1 -> Gain1/1
  delta_F_cmd/1 -> Mux4/1
  delta_y/1 -> Gain3/1, Mux4/2
  Integrator/1 -> Gain2/1
  Mux4/1 -> Kalman_observer/1
  Sum4/1 -> F_cmd_out/1
  delta_alpha/1 -> Mux3/1
  delta_beta/1 -> Mux3/2
  Gain3/1 -> Sum3/2

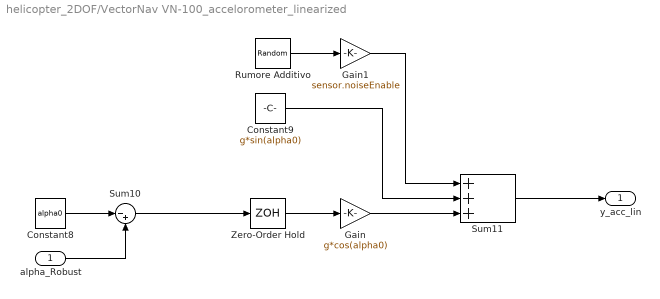
== system helicopter_2DOF/VectorNav VN-100_accelorometer_linearized ==
  alpha_Robust : Inport
  Constant8 : Constant  Value=alpha0
  Constant9 : Constant  Value=g*sin(alpha0)
  Gain : Gain  Gain=g*cos(alpha0)
  Gain1 : Gain  Gain=sensor.noiseEnable
  Rumore Additivo : RandomNumber  Variance=sensor.acc.var  Seed=sensor.seed  SampleTime=sensor.acc.Ts
  Sum10 : Sum  Inputs=|-+
  Sum11 : Sum  Inputs=+++
  Zero-Order Hold : ZeroOrderHold  SampleTime=sensor.acc.Ts
  y_acc_lin : Outport
  wires:
  Zero-Order Hold/1 -> Gain/1
  Constant9/1 -> Sum11/2
  Sum10/1 -> Zero-Order Hold/1
  Rumore Additivo/1 -> Gain1/1
  Gain/1 -> Sum11/3
  Constant8/1 -> Sum10/1
  Sum11/1 -> y_acc_lin/1
  Gain1/1 -> Sum11/1
  alpha_Robust/1 -> Sum10/2

== system helicopter_2DOF/VectorNav VN-100_accelorometer_linearized1 ==
  alpha_Robust : Inport
  Constant8 : Constant  Value=alpha0
  Constant9 : Constant  Value=g*sin(alpha0)
  Gain : Gain  Gain=g*cos(alpha0)
  Gain1 : Gain  Gain=sensor.noiseEnable
  Rumore Additivo : RandomNumber  Variance=sensor.acc.var  Seed=sensor.seed  SampleTime=sensor.acc.Ts
  Sum10 : Sum  Inputs=|-+
  Sum11 : Sum  Inputs=+++
  Zero-Order Hold : ZeroOrderHold  SampleTime=sensor.acc.Ts
  y_acc_lin : Outport
  wires:
  Zero-Order Hold/1 -> Gain/1
  Constant9/1 -> Sum11/2
  Sum10/1 -> Zero-Order Hold/1
  Rumore Additivo/1 -> Gain1/1
  Gain/1 -> Sum11/3
  Constant8/1 -> Sum10/1
  Sum11/1 -> y_acc_lin/1
  Gain1/1 -> Sum11/1
  alpha_Robust/1 -> Sum10/2

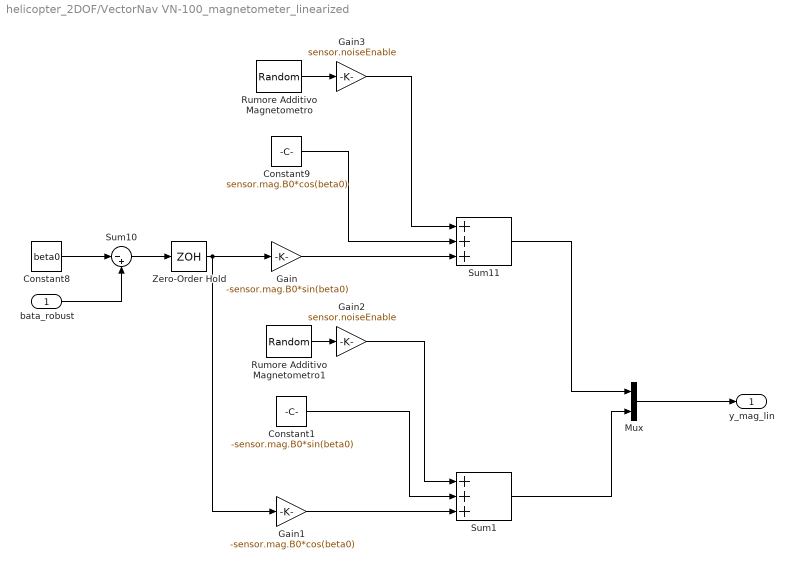
== system helicopter_2DOF/VectorNav VN-100_magnetometer_linearized ==
  bata_robust : Inport
  Constant1 : Constant  Value=-sensor.mag.B0*sin(beta0)
  Constant8 : Constant  Value=beta0
  Constant9 : Constant  Value=sensor.mag.B0*cos(beta0)
  Gain : Gain  Gain=-sensor.mag.B0*sin(beta0)
  Gain1 : Gain  Gain=-sensor.mag.B0*cos(beta0)
  Gain2 : Gain  Gain=sensor.noiseEnable
  Gain3 : Gain  Gain=sensor.noiseEnable
  Mux : Mux  Inputs=2
  Rumore Additivo Magnetometro : RandomNumber  Variance=sensor.mag.var  Seed=sensor.seed + 1  SampleTime=sensor.mag.Ts
  Rumore Additivo Magnetometro1 : RandomNumber  Variance=sensor.mag.var  Seed=sensor.seed + 300  SampleTime=sensor.mag.Ts
  Sum1 : Sum  Inputs=+++
  Sum10 : Sum  Inputs=|-+
  Sum11 : Sum  Inputs=+++
  Zero-Order Hold : ZeroOrderHold  SampleTime=sensor.mag.Ts
  y_mag_lin : Outport
  wires:
  Constant9/1 -> Sum11/2
  Sum10/1 -> Zero-Order Hold/1
  Gain/1 -> Sum11/3
  Constant8/1 -> Sum10/1
  bata_robust/1 -> Sum10/2
  Gain3/1 -> Sum11/1
  Rumore Additivo Magnetometro/1 -> Gain3/1
  Gain1/1 -> Sum1/3
  Constant1/1 -> Sum1/2
  Zero-Order Hold/1 -> Gain/1, Gain1/1
  Rumore Additivo Magnetometro1/1 -> Gain2/1
  Gain2/1 -> Sum1/1
  Sum11/1 -> Mux/1
  Sum1/1 -> Mux/2
  Mux/1 -> y_mag_lin/1

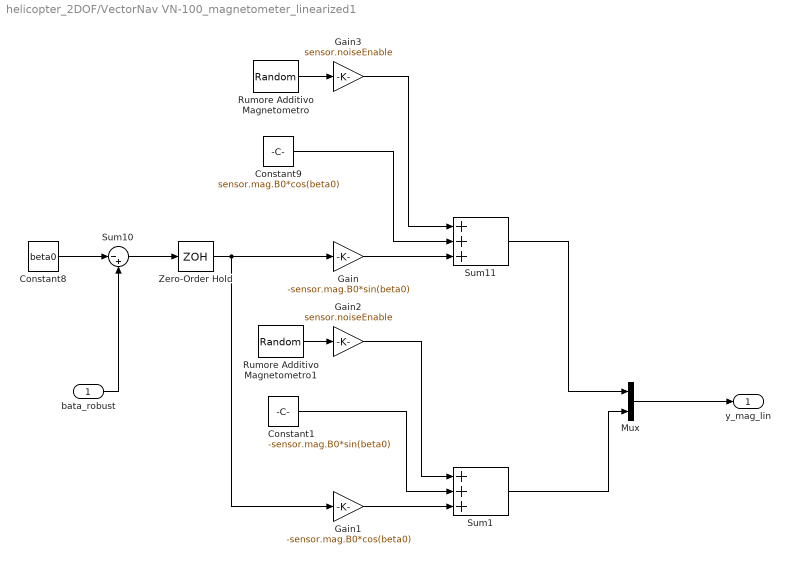
== system helicopter_2DOF/VectorNav VN-100_magnetometer_linearized1 ==
  bata_robust : Inport
  Constant1 : Constant  Value=-sensor.mag.B0*sin(beta0)
  Constant8 : Constant  Value=beta0
  Constant9 : Constant  Value=sensor.mag.B0*cos(beta0)
  Gain : Gain  Gain=-sensor.mag.B0*sin(beta0)
  Gain1 : Gain  Gain=-sensor.mag.B0*cos(beta0)
  Gain2 : Gain  Gain=sensor.noiseEnable
  Gain3 : Gain  Gain=sensor.noiseEnable
  Mux : Mux  Inputs=2
  Rumore Additivo Magnetometro : RandomNumber  Variance=sensor.mag.var  Seed=sensor.seed + 1  SampleTime=sensor.mag.Ts
  Rumore Additivo Magnetometro1 : RandomNumber  Variance=sensor.mag.var  Seed=sensor.seed + 300  SampleTime=sensor.mag.Ts
  Sum1 : Sum  Inputs=+++
  Sum10 : Sum  Inputs=|-+
  Sum11 : Sum  Inputs=+++
  Zero-Order Hold : ZeroOrderHold  SampleTime=sensor.mag.Ts
  y_mag_lin : Outport
  wires:
  Constant9/1 -> Sum11/2
  Sum10/1 -> Zero-Order Hold/1
  Gain/1 -> Sum11/3
  Constant8/1 -> Sum10/1
  bata_robust/1 -> Sum10/2
  Gain3/1 -> Sum11/1
  Rumore Additivo Magnetometro/1 -> Gain3/1
  Gain1/1 -> Sum1/3
  Constant1/1 -> Sum1/2
  Zero-Order Hold/1 -> Gain/1, Gain1/1
  Rumore Additivo Magnetometro1/1 -> Gain2/1
  Gain2/1 -> Sum1/1
  Sum11/1 -> Mux/1
  Sum1/1 -> Mux/2
  Mux/1 -> y_mag_lin/1

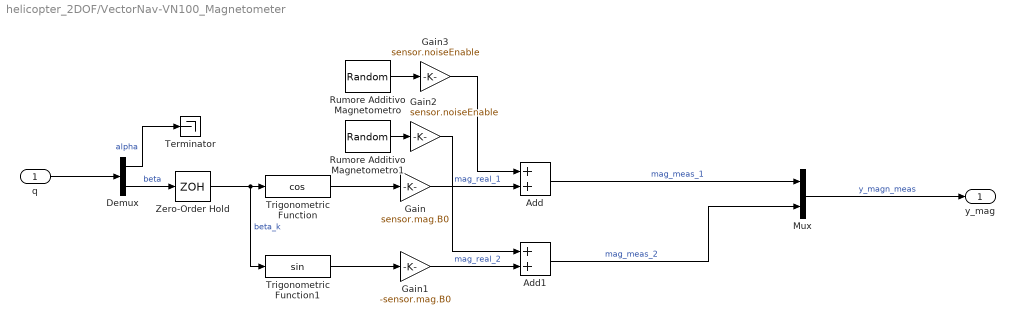
== system helicopter_2DOF/VectorNav-VN100_Magnetometer ==
  q : Inport
  Add : Sum
  Add1 : Sum
  Demux : Demux  Outputs=2
  Gain : Gain  Gain=sensor.mag.B0
  Gain1 : Gain  Gain=-sensor.mag.B0
  Gain2 : Gain  Gain=sensor.noiseEnable
  Gain3 : Gain  Gain=sensor.noiseEnable
  Mux : Mux  Inputs=2
  Rumore Additivo Magnetometro : RandomNumber  Variance=sensor.mag.var  Seed=sensor.seed + 1  SampleTime=sensor.mag.Ts
  Rumore Additivo Magnetometro1 : RandomNumber  Variance=sensor.mag.var  Seed=sensor.seed + 300  SampleTime=sensor.mag.Ts
  Terminator : Terminator
  Trigonometric Function : Trigonometry  Operator=cos
  Trigonometric Function1 : Trigonometry
  Zero-Order Hold : ZeroOrderHold  SampleTime=sensor.mag.Ts
  y_mag : Outport
  wires:
  q/1 -> Demux/1
  Demux/2 -> Zero-Order Hold/1  "beta"
  Demux/1 -> Terminator/1  "alpha"
  Trigonometric Function/1 -> Gain/1
  Trigonometric Function1/1 -> Gain1/1
  Gain/1 -> Add/2  "mag_real_1"
  Rumore Additivo Magnetometro/1 -> Gain3/1
  Gain1/1 -> Add1/2  "mag_real_2"
  Zero-Order Hold/1 -> Trigonometric Function1/1, Trigonometric Function/1  "beta_k"
  Mux/1 -> y_mag/1  "y_magn_meas"
  Add/1 -> Mux/1  "mag_meas_1"
  Rumore Additivo Magnetometro1/1 -> Gain2/1
  Add1/1 -> Mux/2  "mag_meas_2"
  Gain3/1 -> Add/1
  Gain2/1 -> Add1/1

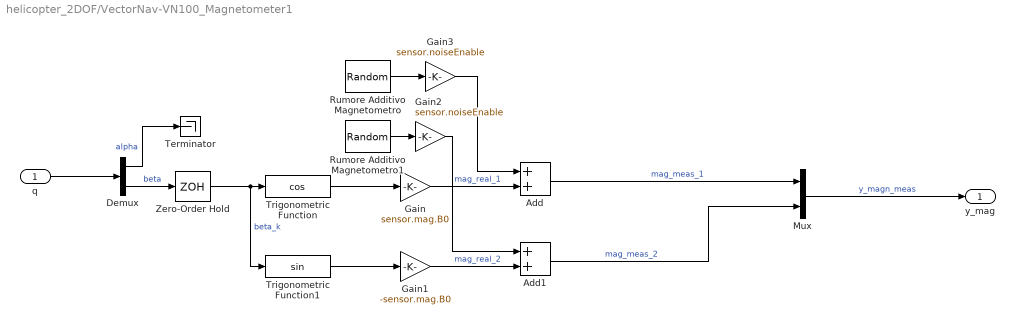
== system helicopter_2DOF/VectorNav-VN100_Magnetometer1 ==
  q : Inport
  Add : Sum
  Add1 : Sum
  Demux : Demux  Outputs=2
  Gain : Gain  Gain=sensor.mag.B0
  Gain1 : Gain  Gain=-sensor.mag.B0
  Gain2 : Gain  Gain=sensor.noiseEnable
  Gain3 : Gain  Gain=sensor.noiseEnable
  Mux : Mux  Inputs=2
  Rumore Additivo Magnetometro : RandomNumber  Variance=sensor.mag.var  Seed=sensor.seed + 1  SampleTime=sensor.mag.Ts
  Rumore Additivo Magnetometro1 : RandomNumber  Variance=sensor.mag.var  Seed=sensor.seed + 300  SampleTime=sensor.mag.Ts
  Terminator : Terminator
  Trigonometric Function : Trigonometry  Operator=cos
  Trigonometric Function1 : Trigonometry
  Zero-Order Hold : ZeroOrderHold  SampleTime=sensor.mag.Ts
  y_mag : Outport
  wires:
  q/1 -> Demux/1
  Demux/2 -> Zero-Order Hold/1  "beta"
  Demux/1 -> Terminator/1  "alpha"
  Trigonometric Function/1 -> Gain/1
  Trigonometric Function1/1 -> Gain1/1
  Gain/1 -> Add/2  "mag_real_1"
  Rumore Additivo Magnetometro/1 -> Gain3/1
  Gain1/1 -> Add1/2  "mag_real_2"
  Zero-Order Hold/1 -> Trigonometric Function1/1, Trigonometric Function/1  "beta_k"
  Mux/1 -> y_mag/1  "y_magn_meas"
  Add/1 -> Mux/1  "mag_meas_1"
  Rumore Additivo Magnetometro1/1 -> Gain2/1
  Add1/1 -> Mux/2  "mag_meas_2"
  Gain3/1 -> Add/1
  Gain2/1 -> Add1/1

== system helicopter_2DOF/VectorNav-VN100_accelerometer ==
  q : Inport
  Add : Sum
  Demux : Demux  Outputs=2
  Gain : Gain  Gain=params.g
  Gain1 : Gain  Gain=sensor.noiseEnable
  Rumore Additivo : RandomNumber  Variance=sensor.acc.var  Seed=sensor.seed  SampleTime=sensor.acc.Ts
  Terminator : Terminator
  Trigonometric Function : Trigonometry
  Zero-Order Hold : ZeroOrderHold  SampleTime=sensor.acc.Ts
  y_acc : Outport
  wires:
  q/1 -> Demux/1
  Demux/1 -> Zero-Order Hold/1  "alpha"
  Demux/2 -> Terminator/1  "beta"
  Trigonometric Function/1 -> Gain/1
  Gain/1 -> Add/2  "real_acc"
  Rumore Additivo/1 -> Gain1/1
  Add/1 -> y_acc/1  "meas_acc"
  Zero-Order Hold/1 -> Trigonometric Function/1  "alpha_k"
  Gain1/1 -> Add/1

== system helicopter_2DOF/VectorNav-VN100_accelerometer1 ==
  q : Inport
  Add : Sum
  Demux : Demux  Outputs=2
  Gain : Gain  Gain=params.g
  Gain1 : Gain  Gain=sensor.noiseEnable
  Rumore Additivo : RandomNumber  Variance=sensor.acc.var  Seed=sensor.seed  SampleTime=sensor.acc.Ts
  Terminator : Terminator
  Trigonometric Function : Trigonometry
  Zero-Order Hold : ZeroOrderHold  SampleTime=sensor.acc.Ts
  y_acc : Outport
  wires:
  q/1 -> Demux/1
  Demux/1 -> Zero-Order Hold/1  "alpha"
  Demux/2 -> Terminator/1  "beta"
  Trigonometric Function/1 -> Gain/1
  Gain/1 -> Add/2  "real_acc"
  Rumore Additivo/1 -> Gain1/1
  Add/1 -> y_acc/1  "meas_acc"
  Zero-Order Hold/1 -> Trigonometric Function/1  "alpha_k"
  Gain1/1 -> Add/1

== system helicopter_2DOF/linearized_2DOF_helicopter_model ==
  delta_F : Inport
  d : Inport  Port=2
  Constant : Constant  Value=x0
  Mux : Mux  Inputs=2
  Sum : Sum  Inputs=|++
  Uncertain State Space : RCTblocks/Uncertain State Space  Tag=USS  USystem=ss(P_nominal_ext.A, P_nominal_ext.B, eye(4), zeros(4,4))  UValue=[]  X0=zeros(4,1)  uX0=[]
  x : Outport
  wires:
  Uncertain State Space/1 -> Sum/1
  Constant/1 -> Sum/2
  Sum/1 -> x/1  "x_linear"
  delta_F/1 -> Mux/1
  d/1 -> Mux/2
  Mux/1 -> Uncertain State Space/1

== system helicopter_2DOF/linearized_2DOF_helicopter_model1 ==
  delta_F : Inport
  d : Inport  Port=2
  Constant : Constant  Value=x0
  Mux : Mux  Inputs=2
  Sum : Sum  Inputs=|++
  Uncertain State Space : RCTblocks/Uncertain State Space  Tag=USS  USystem=ss(P_nominal_ext.A, P_nominal_ext.B, eye(4), zeros(4,4))  UValue=[]  X0=zeros(4,1)  uX0=[]
  x : Outport
  wires:
  Uncertain State Space/1 -> Sum/1
  Constant/1 -> Sum/2
  Sum/1 -> x/1  "x_linear"
  delta_F/1 -> Mux/1
  d/1 -> Mux/2
  Mux/1 -> Uncertain State Space/1

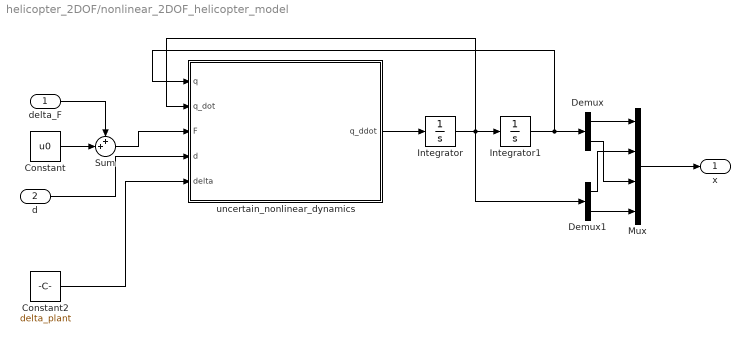
== system helicopter_2DOF/nonlinear_2DOF_helicopter_model ==
  delta_F : Inport
  d : Inport  Port=2
  Constant : Constant  Value=u0
  Constant2 : Constant  Value=delta_plant
  Demux : Demux  Outputs=2
  Demux1 : Demux  Outputs=2
  Integrator : Integrator  InitialCondition=qdot0
  Integrator1 : Integrator  InitialCondition=q0
  Mux : Mux
  Sum : Sum  Inputs=++|
  uncertain_nonlinear_dynamics : MATLAB Function  TreatAsAtomicUnit=on
  x : Outport
  wires:
  Demux1/1 -> Mux/2
  Sum/1 -> uncertain_nonlinear_dynamics/3(F)
  Constant2/1 -> uncertain_nonlinear_dynamics/5(delta)
  Mux/1 -> x/1
  Demux/1 -> Mux/1
  Integrator1/1 -> uncertain_nonlinear_dynamics/1(q), Demux/1
  Demux1/2 -> Mux/4
  uncertain_nonlinear_dynamics/1(q_ddot) -> Integrator/1
  Integrator/1 -> uncertain_nonlinear_dynamics/2(q_dot), Integrator1/1, Demux1/1
  Demux/2 -> Mux/3
  delta_F/1 -> Sum/1
  Constant/1 -> Sum/2
  d/1 -> uncertain_nonlinear_dynamics/4(d)

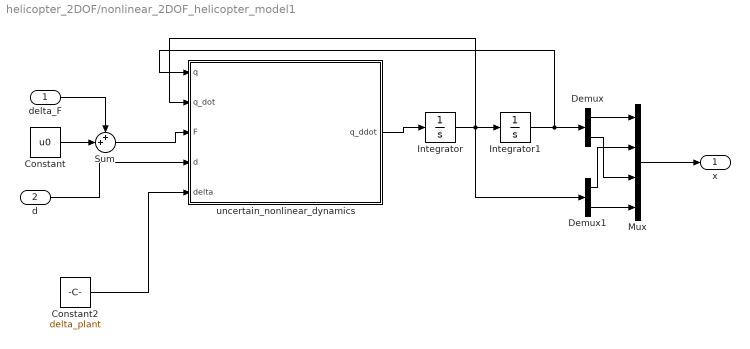
== system helicopter_2DOF/nonlinear_2DOF_helicopter_model1 ==
  delta_F : Inport
  d : Inport  Port=2
  Constant : Constant  Value=u0
  Constant2 : Constant  Value=delta_plant
  Demux : Demux  Outputs=2
  Demux1 : Demux  Outputs=2
  Integrator : Integrator  InitialCondition=qdot0
  Integrator1 : Integrator  InitialCondition=q0
  Mux : Mux
  Sum : Sum  Inputs=++|
  uncertain_nonlinear_dynamics : MATLAB Function  TreatAsAtomicUnit=on
  x : Outport
  wires:
  Demux1/1 -> Mux/2
  Sum/1 -> uncertain_nonlinear_dynamics/3(F)
  Constant2/1 -> uncertain_nonlinear_dynamics/5(delta)
  Mux/1 -> x/1
  Demux/1 -> Mux/1
  Integrator1/1 -> uncertain_nonlinear_dynamics/1(q), Demux/1
  Demux1/2 -> Mux/4
  uncertain_nonlinear_dynamics/1(q_ddot) -> Integrator/1
  Integrator/1 -> uncertain_nonlinear_dynamics/2(q_dot), Integrator1/1, Demux1/1
  Demux/2 -> Mux/3
  delta_F/1 -> Sum/1
  Constant/1 -> Sum/2
  d/1 -> uncertain_nonlinear_dynamics/4(d)

== matlab function helicopter_2DOF/nonlinear_2DOF_helicopter_model1/uncertain_nonlinear_dynamics ==
  data: q input; q_ddot output; q_dot input; F input; d input; delta input
function q_ddot = nonlinear_uncertain_dynamics(q, q_dot, F, d, delta)

    p0.J_alpha = 0.012;       % kg m^2
    p0.J_y = 0.00023;         % kg m^2
    p0.J_z = 0.00364;         % kg m^2
    p0.I_b = 0.00023;         % kg m^2
    
    p0.m = 0.2;               % kg
    p0.l = 0.2;               % m
    
    p0.c_alpha = 0.01;        % N m s/rad
    p0.c_beta  = 0.01;        % N m s/rad
    
    p0.epsilon_p = 0.1;
    p0.epsilon_y = 0.1;
    
    p0.g = 9.81;              % m/s^2
    q_ddot = fcn(q, q_dot, F, d, delta, p0);
end

== matlab function helicopter_2DOF/nonlinear_2DOF_helicopter_model/uncertain_nonlinear_dynamics ==
  data: q input; q_ddot output; q_dot input; F input; d input; delta input
function q_ddot = nonlinear_uncertain_dynamics(q, q_dot, F, d, delta)

    p0.J_alpha = 0.012;       % kg m^2
    p0.J_y = 0.00023;         % kg m^2
    p0.J_z = 0.00364;         % kg m^2
    p0.I_b = 0.00023;         % kg m^2
    
    p0.m = 0.2;               % kg
    p0.l = 0.2;               % m
    
    p0.c_alpha = 0.01;        % N m s/rad
    p0.c_beta  = 0.01;        % N m s/rad
    
    p0.epsilon_p = 0.1;
    p0.epsilon_y = 0.1;
    
    p0.g = 9.81;              % m/s^2
    q_ddot = fcn(q, q_dot, F, d, delta, p0);
end
